simulink model "H2DFRL_LExCI_env"  (R2023a)
settings: Solver=FixedStepAuto  StartTime=0.0  StopTime=50  FixedStep=0.08  RelTol=1e-3
values from neighbouring files (symbols this model uses):
  action_mean_selector_ppo = 1:num_actions    [ReinforcementLearningBlockInit_H2DFRL.m]
  action_sampling_mode = 1    [ReinforcementLearningBlockInit_H2DFRL.m]
  action_selector_ddpg = 1:num_actions    [ReinforcementLearningBlockInit_H2DFRL.m]
  action_std_selector_ppo = 1:num_actions    [ReinforcementLearningBlockInit_H2DFRL.m]
  action_type = 1    [ReinforcementLearningBlockInit_H2DFRL.m]
  C2C_NMPC = init_C2C_NMPC_H2DF(C2C_NMPC.expdata)    [init_H2DFRL_GRU.m]
  LowerLimit = ([0.17e-3;350;-1;1.5e-3] - C2C_NMPC.Normalization.controls.mean)./(C2C_NMPC.Normalization.controls.std)    [init_H2DFRL_GRU.m]
  num_actions = 4    [ReinforcementLearningBlockInit_H2DFRL.m]
  rl_algorithm = 2    [ReinforcementLearningBlockInit_H2DFRL.m]
  Ts = 0.08    [init_H2DFRL_GRU.m]
  UpperLimit = ([0.5e-3;900;0;5.5e-3] - C2C_NMPC.Normalization.controls.mean)./(C2C_NMPC.Normalization.controls.std)    [init_H2DFRL_GRU.m]
undefined symbols (not defined in the file or in its folder): CA50_offset, DiscIntNeverNeededParam, enable_CA50_noise, enable_CA50_offset, enable_IMEP_noise, enable_IMEP_offset, IMEP_offset, NUMBER_OF_ACTIONS
libraries: simulink x15, dspsrcs4 x4, slctrlblks x2, statsLibrary x1
(part 4 of 4)

== system H2DFRL_LExCI_env/Signal Processing/calculate reward/Subsystem/Subsystem1 ==
  UpperBound : Inport
  Lowerbound : Inport  Port=2
  Inputvalue : Inport  Port=3
  AND : Logic  IconShape=distinctive  AllPortsSameDT=off  OutDataTypeStr=boolean
  AND1 : Logic  IconShape=distinctive  AllPortsSameDT=off  OutDataTypeStr=boolean
  Check Dynamic Range : simulink/Model Verification/Check  Dynamic Range  Description=min < u < max  enabled=off  stopWhenAssertionFail=on  export=on  icon=graphic
  Constant2 : Constant  Value=0
  Constant4 : Constant  Value=0
  Gain4 : Gain
  Gain5 : Gain  Gain=0.5
  Gain6 : Gain  Gain=0.5
  GreaterThan : RelationalOperator  Operator=>  OutDataTypeStr=boolean  RndMeth=Simplest  InputSameDT=off
  GreaterThan1 : RelationalOperator  Operator=>  OutDataTypeStr=boolean  RndMeth=Simplest  InputSameDT=off
  NOT : Logic  Operator=NOT  IconShape=distinctive  AllPortsSameDT=off  OutDataTypeStr=boolean
  NOT1 : Logic  Operator=NOT  IconShape=distinctive  AllPortsSameDT=off  OutDataTypeStr=boolean
  Product{,1..3} (4 alike) : Product
  Subtract : Sum  Inputs=+-
  Subtract1 : Sum  Inputs=+-
  Sum : Sum  Inputs=|+++
  Outputvalue : Outport
  wires:
  NOT1/1 -> AND1/2, AND/1
  Product3/1 -> Gain6/1
  Inputvalue/1 -> Check Dynamic Range/3, Subtract/1, Subtract1/2
  Lowerbound/1 -> Subtract1/1, Check Dynamic Range/2
  Gain6/1 -> Sum/3
  AND/1 -> Product3/2
  Gain5/1 -> Sum/2
  UpperBound/1 -> Subtract/2, Check Dynamic Range/1
  Subtract/1 -> Product/1, GreaterThan/1
  Gain4/1 -> Sum/1
  Product/1 -> Product2/1, AND1/1
  Constant2/1 -> GreaterThan/2
  Check Dynamic Range/1 -> NOT/1, NOT1/1
  AND1/1 -> Product2/2
  Product1/1 -> Product3/1, AND/2
  Product2/1 -> Gain5/1
  Subtract1/1 -> Product1/2, GreaterThan1/1
  Constant4/1 -> GreaterThan1/2
  NOT/1 -> Gain4/1
  Sum/1 -> Outputvalue/1
  GreaterThan1/1 -> Product1/1
  GreaterThan/1 -> Product/2

== system H2DFRL_LExCI_env/Signal Processing/calculate reward/Subsystem/Subsystem2 ==
  UpperBound : Inport
  Lowerbound : Inport  Port=2
  Inputvalue : Inport  Port=3
  AND : Logic  IconShape=distinctive  AllPortsSameDT=off  OutDataTypeStr=boolean
  AND1 : Logic  IconShape=distinctive  AllPortsSameDT=off  OutDataTypeStr=boolean
  Check Dynamic Range : simulink/Model Verification/Check  Dynamic Range  Description=min < u < max  enabled=off  stopWhenAssertionFail=on  export=on  icon=graphic
  Constant2 : Constant  Value=0
  Constant4 : Constant  Value=0
  Gain4 : Gain
  Gain5 : Gain  Gain=0.5
  Gain6 : Gain  Gain=0.5
  GreaterThan : RelationalOperator  Operator=>  OutDataTypeStr=boolean  RndMeth=Simplest  InputSameDT=off
  GreaterThan1 : RelationalOperator  Operator=>  OutDataTypeStr=boolean  RndMeth=Simplest  InputSameDT=off
  NOT : Logic  Operator=NOT  IconShape=distinctive  AllPortsSameDT=off  OutDataTypeStr=boolean
  NOT1 : Logic  Operator=NOT  IconShape=distinctive  AllPortsSameDT=off  OutDataTypeStr=boolean
  Product{,1..3} (4 alike) : Product
  Subtract : Sum  Inputs=+-
  Subtract1 : Sum  Inputs=+-
  Sum : Sum  Inputs=|+++
  Outputvalue : Outport
  wires:
  NOT1/1 -> AND1/2, AND/1
  Product3/1 -> Gain6/1
  Inputvalue/1 -> Check Dynamic Range/3, Subtract/1, Subtract1/2
  Lowerbound/1 -> Subtract1/1, Check Dynamic Range/2
  Gain6/1 -> Sum/3
  AND/1 -> Product3/2
  Gain5/1 -> Sum/2
  UpperBound/1 -> Subtract/2, Check Dynamic Range/1
  Subtract/1 -> Product/1, GreaterThan/1
  Gain4/1 -> Sum/1
  Product/1 -> Product2/1, AND1/1
  Constant2/1 -> GreaterThan/2
  Check Dynamic Range/1 -> NOT/1, NOT1/1
  AND1/1 -> Product2/2
  Product1/1 -> Product3/1, AND/2
  Product2/1 -> Gain5/1
  Subtract1/1 -> Product1/2, GreaterThan1/1
  Constant4/1 -> GreaterThan1/2
  NOT/1 -> Gain4/1
  Sum/1 -> Outputvalue/1
  GreaterThan1/1 -> Product1/1
  GreaterThan/1 -> Product/2

== system H2DFRL_LExCI_env/Signal Processing/calculate reward/Subsystem/Subsystem3 ==
  UpperBound : Inport
  Lowerbound : Inport  Port=2
  Inputvalue : Inport  Port=3
  AND : Logic  IconShape=distinctive  AllPortsSameDT=off  OutDataTypeStr=boolean
  AND1 : Logic  IconShape=distinctive  AllPortsSameDT=off  OutDataTypeStr=boolean
  Check Dynamic Range : simulink/Model Verification/Check  Dynamic Range  Description=min < u < max  enabled=off  stopWhenAssertionFail=on  export=on  icon=graphic
  Constant2 : Constant  Value=0
  Constant4 : Constant  Value=0
  Gain4 : Gain
  Gain5 : Gain  Gain=0.5
  Gain6 : Gain  Gain=0.5
  GreaterThan : RelationalOperator  Operator=>  OutDataTypeStr=boolean  RndMeth=Simplest  InputSameDT=off
  GreaterThan1 : RelationalOperator  Operator=>  OutDataTypeStr=boolean  RndMeth=Simplest  InputSameDT=off
  NOT : Logic  Operator=NOT  IconShape=distinctive  AllPortsSameDT=off  OutDataTypeStr=boolean
  NOT1 : Logic  Operator=NOT  IconShape=distinctive  AllPortsSameDT=off  OutDataTypeStr=boolean
  Product{,1..3} (4 alike) : Product
  Subtract : Sum  Inputs=+-
  Subtract1 : Sum  Inputs=+-
  Sum : Sum  Inputs=|+++
  Outputvalue : Outport
  wires:
  NOT1/1 -> AND1/2, AND/1
  Product3/1 -> Gain6/1
  Inputvalue/1 -> Check Dynamic Range/3, Subtract/1, Subtract1/2
  Lowerbound/1 -> Subtract1/1, Check Dynamic Range/2
  Gain6/1 -> Sum/3
  AND/1 -> Product3/2
  Gain5/1 -> Sum/2
  UpperBound/1 -> Subtract/2, Check Dynamic Range/1
  Subtract/1 -> Product/1, GreaterThan/1
  Gain4/1 -> Sum/1
  Product/1 -> Product2/1, AND1/1
  Constant2/1 -> GreaterThan/2
  Check Dynamic Range/1 -> NOT/1, NOT1/1
  AND1/1 -> Product2/2
  Product1/1 -> Product3/1, AND/2
  Product2/1 -> Gain5/1
  Subtract1/1 -> Product1/2, GreaterThan1/1
  Constant4/1 -> GreaterThan1/2
  NOT/1 -> Gain4/1
  Sum/1 -> Outputvalue/1
  GreaterThan1/1 -> Product1/1
  GreaterThan/1 -> Product/2

== system H2DFRL_LExCI_env/Signal Processing/calculate reward/Subsystem/Subsystem4 ==
  UpperBound : Inport
  Lowerbound : Inport  Port=2
  Inputvalue : Inport  Port=3
  AND : Logic  IconShape=distinctive  AllPortsSameDT=off  OutDataTypeStr=boolean
  AND1 : Logic  IconShape=distinctive  AllPortsSameDT=off  OutDataTypeStr=boolean
  Check Dynamic Range : simulink/Model Verification/Check  Dynamic Range  Description=min < u < max  enabled=off  stopWhenAssertionFail=on  export=on  icon=graphic
  Constant2 : Constant  Value=0
  Constant4 : Constant  Value=0
  Gain4 : Gain
  Gain5 : Gain  Gain=0.5
  Gain6 : Gain  Gain=0.5
  GreaterThan : RelationalOperator  Operator=>  OutDataTypeStr=boolean  RndMeth=Simplest  InputSameDT=off
  GreaterThan1 : RelationalOperator  Operator=>  OutDataTypeStr=boolean  RndMeth=Simplest  InputSameDT=off
  NOT : Logic  Operator=NOT  IconShape=distinctive  AllPortsSameDT=off  OutDataTypeStr=boolean
  NOT1 : Logic  Operator=NOT  IconShape=distinctive  AllPortsSameDT=off  OutDataTypeStr=boolean
  Product{,1..3} (4 alike) : Product
  Subtract : Sum  Inputs=+-
  Subtract1 : Sum  Inputs=+-
  Sum : Sum  Inputs=|+++
  Outputvalue : Outport
  wires:
  NOT1/1 -> AND1/2, AND/1
  Product3/1 -> Gain6/1
  Inputvalue/1 -> Check Dynamic Range/3, Subtract/1, Subtract1/2
  Lowerbound/1 -> Subtract1/1, Check Dynamic Range/2
  Gain6/1 -> Sum/3
  AND/1 -> Product3/2
  Gain5/1 -> Sum/2
  UpperBound/1 -> Subtract/2, Check Dynamic Range/1
  Subtract/1 -> Product/1, GreaterThan/1
  Gain4/1 -> Sum/1
  Product/1 -> Product2/1, AND1/1
  Constant2/1 -> GreaterThan/2
  Check Dynamic Range/1 -> NOT/1, NOT1/1
  AND1/1 -> Product2/2
  Product1/1 -> Product3/1, AND/2
  Product2/1 -> Gain5/1
  Subtract1/1 -> Product1/2, GreaterThan1/1
  Constant4/1 -> GreaterThan1/2
  NOT/1 -> Gain4/1
  Sum/1 -> Outputvalue/1
  GreaterThan1/1 -> Product1/1
  GreaterThan/1 -> Product/2

== system H2DFRL_LExCI_env/Signal Processing/calculate reward/Subsystem/Subsystem5 ==
  inputValue : Inport
  Add14 : Sum
  Multiply31 : Product
  Multiply32 : Product
  Multiply4 : Product
  Tanh3 : Trigonometry  Operator=tanh
  mcrl_fRwrdIMEPTracking_C1 : Constant  Value=3
  mcrl_fRwrdIMEPTracking_C2 : Constant  Value=1.5
  mcrl_fRwrdIMEPTracking_C3 : Constant  Value=0.1
  outValue : Outport
  wires:
  mcrl_fRwrdIMEPTracking_C1/1 -> Multiply32/2
  inputValue/1 -> Multiply31/1, Multiply32/1
  Multiply31/1 -> Add14/1
  mcrl_fRwrdIMEPTracking_C2/1 -> Multiply4/2
  Multiply32/1 -> Tanh3/1
  mcrl_fRwrdIMEPTracking_C3/1 -> Multiply31/2
  Add14/1 -> outValue/1
  Tanh3/1 -> Multiply4/1
  Multiply4/1 -> Add14/2

== system H2DFRL_LExCI_env/Signal Processing/calculate reward/Subsystem/Subsystem6 ==
  inputValue : Inport
  Add14 : Sum
  Multiply31 : Product
  Multiply32 : Product
  Multiply4 : Product
  Tanh3 : Trigonometry  Operator=tanh
  mcrl_fRwrdIMEPTracking_C1 : Constant  Value=3
  mcrl_fRwrdIMEPTracking_C2 : Constant  Value=1.5
  mcrl_fRwrdIMEPTracking_C3 : Constant  Value=0.1
  outValue : Outport
  wires:
  mcrl_fRwrdIMEPTracking_C1/1 -> Multiply32/2
  inputValue/1 -> Multiply31/1, Multiply32/1
  Multiply31/1 -> Add14/1
  mcrl_fRwrdIMEPTracking_C2/1 -> Multiply4/2
  Multiply32/1 -> Tanh3/1
  mcrl_fRwrdIMEPTracking_C3/1 -> Multiply31/2
  Add14/1 -> outValue/1
  Tanh3/1 -> Multiply4/1
  Multiply4/1 -> Add14/2

== system H2DFRL_LExCI_env/Signal Processing/calculate reward/Subsystem/TrackingError ==
  Outputs : Inport
  ReferenceOutputs : Inport  Port=2
  Demux1 : Demux
  Demux2 : Demux
  Mux : Mux
  Subtract{,1..3} (4 alike) : Sum  Inputs=+-
  TrackingError : Outport
  wires:
  Demux2/4 -> Subtract3/2
  Demux1/2 -> Subtract1/1
  Demux1/1 -> Subtract/1
  Demux2/2 -> Subtract1/2
  Demux2/3 -> Subtract2/2
  Outputs/1 -> Demux2/1
  Demux1/3 -> Subtract2/1
  Demux1/4 -> Subtract3/1
  Demux2/1 -> Subtract/2
  Mux/1 -> TrackingError/1
  Subtract/1 -> Mux/1
  Subtract1/1 -> Mux/2
  Subtract2/1 -> Mux/3
  Subtract3/1 -> Mux/4
  ReferenceOutputs/1 -> Demux1/1

== system H2DFRL_LExCI_env/RL_Block/RL_Agent/Sampling/Continuous Action/DDPG_Sampler ==
  norm_action_dist : Inport
  b_training_active : Inport  Port=2
  standard_deviation : Inport  Port=3
  Action Selector1 : Constant  Value=action_selector_ddpg  OutDataTypeStr=single
  Add : Sum
  Constant : Constant  Value=0  OutDataTypeStr=single
  Data Type Conversion : DataTypeConversion  OutDataTypeStr=single  SaturateOnIntegerOverflow=off  RndMeth=Floor
  Divide : Product  Inputs=**
  Random Number : RandomNumber  Mean=zeros(1,num_actions)  Variance=ones(1,num_actions)  Seed=1732920383
  Selector : Selector  IndexOptions=Index vector (port)  Indices=1  OutputSizes=1
  Switch : Switch  Criteria=u2 > Threshold  SaturateOnIntegerOverflow=off  InputSameDT=off
  "norm_action " : Outport
  wires:
  Switch/1 -> Divide/2
  standard_deviation/1 -> Divide/1
  b_training_active/1 -> Switch/2
  Constant/1 -> Switch/3
  Random Number/1 -> Data Type Conversion/1
  Add/1 -> "norm_action "/1
  Data Type Conversion/1 -> Switch/1
  norm_action_dist/1 -> Selector/1
  Divide/1 -> Add/2
  Action Selector1/1 -> Selector/2
  Selector/1 -> Add/1

== system H2DFRL_LExCI_env/RL_Block/RL_Agent/Sampling/Continuous Action/PPO_Sampler ==
  norm_action_dist : Inport
  b_training_active : Inport  Port=2
  Action Mean Selector : Constant  Value=action_mean_selector_ppo  OutDataTypeStr=single
  Action Std Selector : Constant  Value=action_std_selector_ppo  OutDataTypeStr=single
  Add : Sum
  Constant : Constant  Value=0  OutDataTypeStr=single
  Data Type Conversion : DataTypeConversion  OutDataTypeStr=single  SaturateOnIntegerOverflow=off  RndMeth=Floor
  Divide : Product  Inputs=**
  Math Function : Math
  Mean Selector : Selector  IndexOptions=Index vector (port)  Indices=1  OutputSizes=1
  Random Number : RandomNumber  Mean=zeros(1,num_actions)  Variance=ones(1,num_actions)  Seed=1732920383
  StdDev Selector : Selector  IndexOptions=Index vector (port)  Indices=2  OutputSizes=1
  Switch : Switch  Criteria=u2 > Threshold  SaturateOnIntegerOverflow=off  InputSameDT=off
  "norm_action " : Outport
  wires:
  Divide/1 -> Add/2
  Mean Selector/1 -> Add/1
  Data Type Conversion/1 -> Switch/1
  Add/1 -> "norm_action "/1
  StdDev Selector/1 -> Math Function/1
  Random Number/1 -> Data Type Conversion/1
  Action Mean Selector/1 -> Mean Selector/2
  Constant/1 -> Switch/3
  b_training_active/1 -> Switch/2
  Math Function/1 -> Divide/1
  Action Std Selector/1 -> StdDev Selector/2
  Switch/1 -> Divide/2
  norm_action_dist/1 -> StdDev Selector/1, Mean Selector/1

== system H2DFRL_LExCI_env/Signal Processing/calculate reward/Subsystem/Staging/Subsystem ==
  IMEP_norm1 : Inport
  Constant4 : Constant  Value=C2C_NMPC.Normalization.outputs.mean(1)
  Gain2 : Gain  Gain=C2C_NMPC.Normalization.outputs.std(1)
  Sum4 : Sum  Inputs=|++
  IMEP1 : Outport
  wires:
  Sum4/1 -> IMEP1/1
  Constant4/1 -> Sum4/2
  Gain2/1 -> Sum4/1
  IMEP_norm1/1 -> Gain2/1

== system H2DFRL_LExCI_env/Signal Processing/calculate reward/Subsystem/Staging/Subsystem1 ==
  IMEP_norm1 : Inport
  Constant4 : Constant  Value=C2C_NMPC.Normalization.outputs.mean(1)
  Gain2 : Gain  Gain=C2C_NMPC.Normalization.outputs.std(1)
  Sum4 : Sum  Inputs=|++
  IMEP1 : Outport
  wires:
  Sum4/1 -> IMEP1/1
  Constant4/1 -> Sum4/2
  Gain2/1 -> Sum4/1
  IMEP_norm1/1 -> Gain2/1

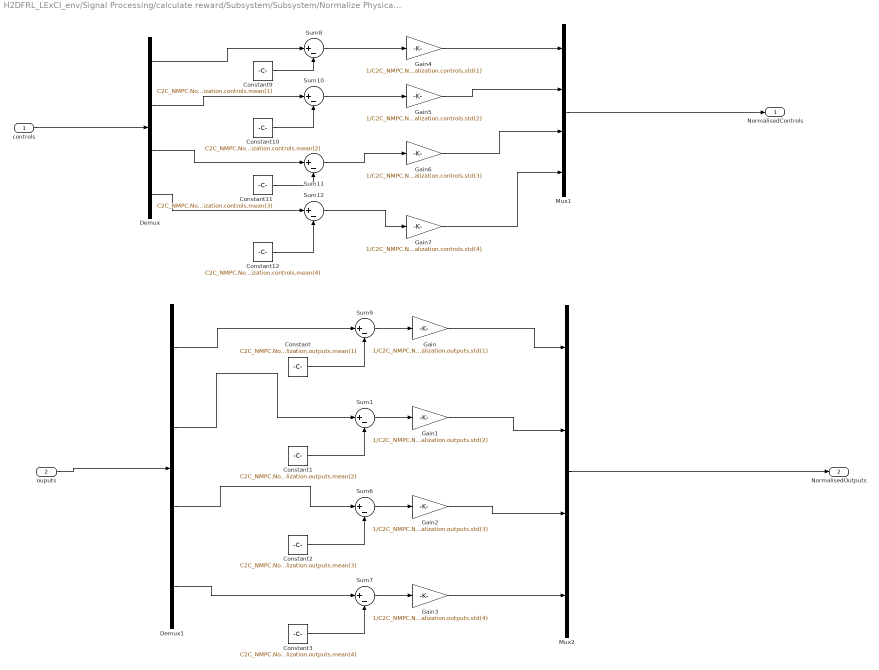
== system H2DFRL_LExCI_env/Signal Processing/calculate reward/Subsystem/Subsystem/Normalize Physical Controls and Outputs2 ==
  controls : Inport
  "ouputs " : Inport  Port=2
  Constant : Constant  Value=C2C_NMPC.Normalization.outputs.mean(1)
  Constant1 : Constant  Value=C2C_NMPC.Normalization.outputs.mean(2)
  Constant10 : Constant  Value=C2C_NMPC.Normalization.controls.mean(2)
  Constant11 : Constant  Value=C2C_NMPC.Normalization.controls.mean(3)
  Constant12 : Constant  Value=C2C_NMPC.Normalization.controls.mean(4)
  Constant2 : Constant  Value=C2C_NMPC.Normalization.outputs.mean(3)
  Constant3 : Constant  Value=C2C_NMPC.Normalization.outputs.mean(4)
  Constant9 : Constant  Value=C2C_NMPC.Normalization.controls.mean(1)
  Demux : Demux
  Demux1 : Demux
  Gain : Gain  Gain=1/C2C_NMPC.Normalization.outputs.std(1)
  Gain1 : Gain  Gain=1/C2C_NMPC.Normalization.outputs.std(2)
  Gain2 : Gain  Gain=1/C2C_NMPC.Normalization.outputs.std(3)
  Gain3 : Gain  Gain=1/C2C_NMPC.Normalization.outputs.std(4)
  Gain4 : Gain  Gain=1/C2C_NMPC.Normalization.controls.std(1)
  Gain5 : Gain  Gain=1/C2C_NMPC.Normalization.controls.std(2)
  Gain6 : Gain  Gain=1/C2C_NMPC.Normalization.controls.std(3)
  Gain7 : Gain  Gain=1/C2C_NMPC.Normalization.controls.std(4)
  Mux1 : Mux
  Mux2 : Mux
  Sum{1,6..12} (8 alike) : Sum  Inputs=|+-
  "NormalisedControls " : Outport
  NormalisedOutputs : Outport  Port=2
  wires:
  Constant2/1 -> Sum6/2
  Gain7/1 -> Mux1/4
  Gain5/1 -> Mux1/2
  Constant12/1 -> Sum12/2
  Constant11/1 -> Sum11/2
  Gain4/1 -> Mux1/1
  Demux/1 -> Sum8/1
  Demux1/2 -> Sum1/1
  Constant/1 -> Sum9/2
  Sum11/1 -> Gain6/1
  Demux/4 -> Sum12/1
  Gain6/1 -> Mux1/3
  Constant1/1 -> Sum1/2
  Demux1/4 -> Sum7/1
  Demux1/3 -> Sum6/1
  Sum6/1 -> Gain2/1
  Sum9/1 -> Gain/1
  Sum10/1 -> Gain5/1
  Mux1/1 -> "NormalisedControls "/1
  Sum8/1 -> Gain4/1
  Sum12/1 -> Gain7/1
  Constant9/1 -> Sum8/2
  Demux/2 -> Sum10/1
  Constant10/1 -> Sum10/2
  Constant3/1 -> Sum7/2
  Sum1/1 -> Gain1/1
  Demux/3 -> Sum11/1
  Sum7/1 -> Gain3/1
  controls/1 -> Demux/1
  "ouputs "/1 -> Demux1/1
  Demux1/1 -> Sum9/1
  Gain1/1 -> Mux2/2
  Gain/1 -> Mux2/1
  Gain2/1 -> Mux2/3
  Gain3/1 -> Mux2/4
  Mux2/1 -> NormalisedOutputs/1

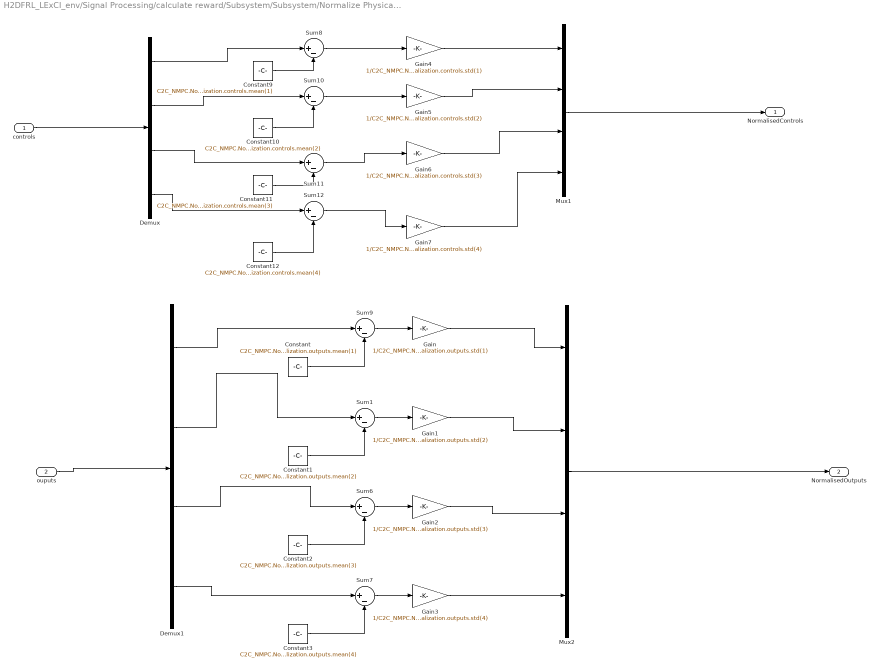
== system H2DFRL_LExCI_env/Signal Processing/calculate reward/Subsystem/Subsystem/Normalize Physical Controls and Outputs3 ==
  controls : Inport
  "ouputs " : Inport  Port=2
  Constant : Constant  Value=C2C_NMPC.Normalization.outputs.mean(1)
  Constant1 : Constant  Value=C2C_NMPC.Normalization.outputs.mean(2)
  Constant10 : Constant  Value=C2C_NMPC.Normalization.controls.mean(2)
  Constant11 : Constant  Value=C2C_NMPC.Normalization.controls.mean(3)
  Constant12 : Constant  Value=C2C_NMPC.Normalization.controls.mean(4)
  Constant2 : Constant  Value=C2C_NMPC.Normalization.outputs.mean(3)
  Constant3 : Constant  Value=C2C_NMPC.Normalization.outputs.mean(4)
  Constant9 : Constant  Value=C2C_NMPC.Normalization.controls.mean(1)
  Demux : Demux
  Demux1 : Demux
  Gain : Gain  Gain=1/C2C_NMPC.Normalization.outputs.std(1)
  Gain1 : Gain  Gain=1/C2C_NMPC.Normalization.outputs.std(2)
  Gain2 : Gain  Gain=1/C2C_NMPC.Normalization.outputs.std(3)
  Gain3 : Gain  Gain=1/C2C_NMPC.Normalization.outputs.std(4)
  Gain4 : Gain  Gain=1/C2C_NMPC.Normalization.controls.std(1)
  Gain5 : Gain  Gain=1/C2C_NMPC.Normalization.controls.std(2)
  Gain6 : Gain  Gain=1/C2C_NMPC.Normalization.controls.std(3)
  Gain7 : Gain  Gain=1/C2C_NMPC.Normalization.controls.std(4)
  Mux1 : Mux
  Mux2 : Mux
  Sum{1,6..12} (8 alike) : Sum  Inputs=|+-
  "NormalisedControls " : Outport
  NormalisedOutputs : Outport  Port=2
  wires:
  Constant2/1 -> Sum6/2
  Gain7/1 -> Mux1/4
  Gain5/1 -> Mux1/2
  Constant12/1 -> Sum12/2
  Constant11/1 -> Sum11/2
  Gain4/1 -> Mux1/1
  Demux/1 -> Sum8/1
  Demux1/2 -> Sum1/1
  Constant/1 -> Sum9/2
  Sum11/1 -> Gain6/1
  Demux/4 -> Sum12/1
  Gain6/1 -> Mux1/3
  Constant1/1 -> Sum1/2
  Demux1/4 -> Sum7/1
  Demux1/3 -> Sum6/1
  Sum6/1 -> Gain2/1
  Sum9/1 -> Gain/1
  Sum10/1 -> Gain5/1
  Mux1/1 -> "NormalisedControls "/1
  Sum8/1 -> Gain4/1
  Sum12/1 -> Gain7/1
  Constant9/1 -> Sum8/2
  Demux/2 -> Sum10/1
  Constant10/1 -> Sum10/2
  Constant3/1 -> Sum7/2
  Sum1/1 -> Gain1/1
  Demux/3 -> Sum11/1
  Sum7/1 -> Gain3/1
  controls/1 -> Demux/1
  "ouputs "/1 -> Demux1/1
  Demux1/1 -> Sum9/1
  Gain1/1 -> Mux2/2
  Gain/1 -> Mux2/1
  Gain2/1 -> Mux2/3
  Gain3/1 -> Mux2/4
  Mux2/1 -> NormalisedOutputs/1

== matlab function H2DFRL_LExCI_env/Engine Model/dyn_H2DF/dyn_H2DF ==
  data: last_LSTM_states input; controls input; outputs output; last_outputs input; H2DF_Par parameter; LSTM_states output
 function [outputs, LSTM_states] = dyn_H2DF(last_LSTM_states, controls, last_outputs, H2DF_Par)

[outputs, LSTM_states] = dyn_H2DF_GRU(last_LSTM_states, [controls; last_outputs(1)], H2DF_Par);

== matlab function H2DFRL_LExCI_env/Engine Model/dyn_H2DF_state_augmentation/dyn_H2DF_state_augmentation ==
  data: last_LSTM_states input; LSTM_states output; controls input; last_outputs input; H2DF_Par parameter
function LSTM_states = dyn_H2DF_state_augmentation(last_LSTM_states, controls, last_outputs, H2DF_Par)

LSTM_states = dyn_H2DF_state_augmentation_GRU(last_LSTM_states,[controls; last_outputs(1)], H2DF_Par);

== matlab function H2DFRL_LExCI_env/references/MATLAB Function ==
  data: t input; IMEP_ref output; rchange1 input; NOx_ref output; SOOT_ref output; MPRR_ref output; DOI_Main_ref output; P2M_ref output; SOI_ref output; DOI_H2_ref output; rchange2 input; rchange3 input; rchange4 input
function [IMEP_ref, NOx_ref, SOOT_ref, MPRR_ref, DOI_Main_ref, P2M_ref, SOI_ref, DOI_H2_ref] = fcn(t, rchange1,rchange2,rchange3,rchange4)
% IMEP_ref =5e5;
% NOx_ref =    66.8796;
% SOOT_ref= 0.2830;
% MPRR_ref= 17416;
% DOI_Main_ref =    1.7005e-04; 
% P2M_ref= 430;
% SOI_ref= -5.9815;
% DOI_H2_ref= 0.0017;

IMEP_ref = 5e5;
NOx_ref = 0;
SOOT_ref= 0;
MPRR_ref= 0;
DOI_Main_ref = 0; 
P2M_ref= 0;
SOI_ref= 0;
DOI_H2_ref= 0;

IMEP_ref = rchange1;
if t>1 && t<7.5
  IMEP_ref = rchange1; %[Outputs, Controls]
 
elseif t>=7.5 && t<15 
  IMEP_ref = rchange1*rchange2;

elseif t>=15  && t<25
  IMEP_ref = rchange1*rchange2*rchange3;

elseif t>=25  && t<30
  IMEP_ref = rchange1*rchange3;

elseif t>=30 && t<35
    IMEP_ref = (1-(t-30)/5)*rchange1*rchange3+((t-30)/5)*rchange1*rchange4; 

elseif t>35 && t<45
    IMEP_ref = rchange1*rchange4;

elseif t>=45 && t<60 
    IMEP_ref = (1-(t-45)/15)*rchange1*rchange4+((t-45)/15)*rchange1*rchange2*rchange3*rchange4;

elseif t>=60  && t<75
    IMEP_ref = rchange1*rchange2*rchange3*rchange4;

elseif t>=75 && t<100 
    IMEP_ref = (1-(t-75)/25)*rchange1*rchange2*rchange3*rchange4+((t-75)/25)*rchange1*rchange2*rchange4;
 
elseif t>=100
    IMEP_ref = rchange1*rchange2*rchange4;

end

if IMEP_ref<3e5
    IMEP_ref = 3e5;
elseif IMEP_ref > 8e5
    IMEP_ref = 8e5;
end

% 
% if t>4
%  IMEP_ref = 0.8*rchange; %[Outputs, Controls]
% end
% if t>5 
%     IMEP_ref = 0.6*rchange;
% end
% if t>6 
%     IMEP_ref = 1.4*rchange;
% end
% if t>7
%  IMEP_ref = rchange; %[Outputs, Controls]
% end
% if t>8 
%     IMEP_ref = 0.4*rchange;
% end
% if t>9 
%     IMEP_ref = 1.1*rchange;
% end
